simulink model "RobotRuka"  (R2020a)
settings: Solver=VariableStepAuto  StartTime=0.0  StopTime=10.0  RelTol=1e-3
values from neighbouring files (symbols this model uses):
  g = 9.81    [Podaci.m]
  Kd = 200    [Podaci.m]
  Kp = 900    [Podaci.m]
  lc1 = 0.8    [Podaci.m]
  m0 = m1*lc1*lc1+Il2    (= 6.5)    [Podaci.m]
  m1 = 10    [Podaci.m]
  m2 = 10    [Podaci.m]
libraries: fuzblock x2
settings Model: Creator=Aldin  LastModifiedBy=Aldin

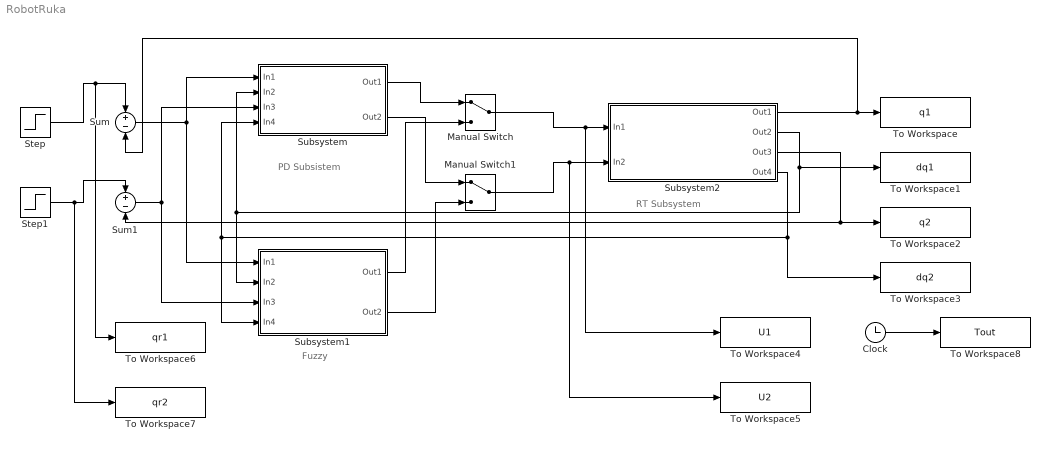
== system RobotRuka ==
  note: PD Subsistem
  note: Fuzzy
  note: RT Subsystem
  Clock : Clock
  Manual Switch : ManualSwitch
  Manual Switch1 : ManualSwitch
  Step : Step  Time=0  SampleTime=0
  Step1 : Step  Time=0  SampleTime=0
  Subsystem : Subsystem
  Subsystem1 : Subsystem
  Subsystem2 : Subsystem
  Sum : Sum  Inputs=+-
  Sum1 : Sum  Inputs=+-
  To Workspace : ToWorkspace  VariableName=q1  SampleTime=-1
  To Workspace1 : ToWorkspace  VariableName=dq1  SampleTime=-1
  To Workspace2 : ToWorkspace  VariableName=q2  SampleTime=-1
  To Workspace3 : ToWorkspace  VariableName=dq2  SampleTime=-1
  To Workspace4 : ToWorkspace  VariableName=U1  SampleTime=-1
  To Workspace5 : ToWorkspace  VariableName=U2  SampleTime=-1
  To Workspace6 : ToWorkspace  VariableName=qr1  SampleTime=-1
  To Workspace7 : ToWorkspace  VariableName=qr2  SampleTime=-1
  To Workspace8 : ToWorkspace  VariableName=Tout  SampleTime=-1
  wires:
  Subsystem2/4(Out4) -> Subsystem/4(In4), Subsystem1/4(In4), To Workspace3/1
  Subsystem1/2(Out2) -> Manual Switch1/2
  Clock/1 -> To Workspace8/1
  Manual Switch/1 -> To Workspace4/1, Subsystem2/1(In1)
  Subsystem2/1(Out1) -> To Workspace/1, Sum/2
  Subsystem1/1(Out1) -> Manual Switch/2
  Subsystem2/3(Out3) -> Sum1/2, To Workspace2/1
  Manual Switch1/1 -> To Workspace5/1, Subsystem2/2(In2)
  Sum1/1 -> Subsystem1/3(In3), Subsystem/3(In3)
  Subsystem2/2(Out2) -> To Workspace1/1, Subsystem1/2(In2), Subsystem/2(In2)
  Step1/1 -> To Workspace7/1, Sum1/1
  Sum/1 -> Subsystem/1(In1), Subsystem1/1(In1)
  Subsystem/1(Out1) -> Manual Switch/1
  Step/1 -> To Workspace6/1, Sum/1
  Subsystem/2(Out2) -> Manual Switch1/1

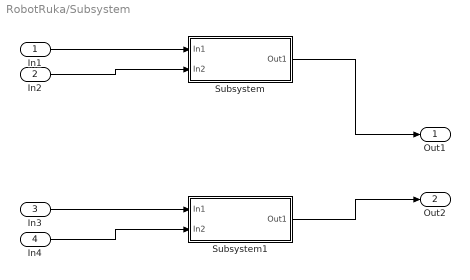
== system RobotRuka/Subsystem ==
  In1 : Inport
  In2 : Inport  Port=2
  In3 : Inport  Port=3
  In4 : Inport  Port=4
  Subsystem : Subsystem
  Subsystem1 : Subsystem
  Out1 : Outport
  Out2 : Outport  Port=2
  wires:
  Subsystem/1(Out1) -> Out1/1
  In1/1 -> Subsystem/1(In1)
  In2/1 -> Subsystem/2(In2)
  In3/1 -> Subsystem1/1(In1)
  In4/1 -> Subsystem1/2(In2)
  Subsystem1/1(Out1) -> Out2/1

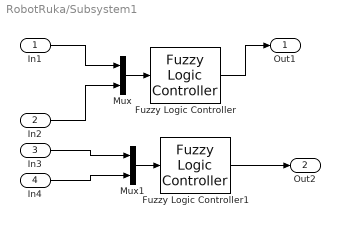
== system RobotRuka/Subsystem1 ==
  In1 : Inport
  In2 : Inport  Port=2
  In3 : Inport  Port=3
  In4 : Inport  Port=4
  Fuzzy Logic Controller : fuzblock/Fuzzy Logic  Controller  FIS=rtfuzzy  OutputSampleNumber=101  DataType=double  FuzzifiedInputs=off  RuleFiringStrengths=off  RuleOutputs=off  AggregatedOutputs=off  SimulateUsing=Interpreted execution  OutOfRangeInputValueMessage=warning  NoRuleFiredMessage=warning  EmptyOutputFuzzySetMessage=warning
  Fuzzy Logic Controller1 : fuzblock/Fuzzy Logic  Controller  FIS=rtfuzzy  OutputSampleNumber=101  DataType=double  FuzzifiedInputs=off  RuleFiringStrengths=off  RuleOutputs=off  AggregatedOutputs=off  SimulateUsing=Interpreted execution  OutOfRangeInputValueMessage=warning  NoRuleFiredMessage=warning  EmptyOutputFuzzySetMessage=warning
  Mux : Mux  Inputs=2
  Mux1 : Mux  Inputs=2
  Out1 : Outport
  Out2 : Outport  Port=2
  wires:
  Mux/1 -> Fuzzy Logic Controller/1
  In1/1 -> Mux/1
  In2/1 -> Mux/2
  Fuzzy Logic Controller/1 -> Out1/1
  Mux1/1 -> Fuzzy Logic Controller1/1
  In3/1 -> Mux1/1
  In4/1 -> Mux1/2
  Fuzzy Logic Controller1/1 -> Out2/1

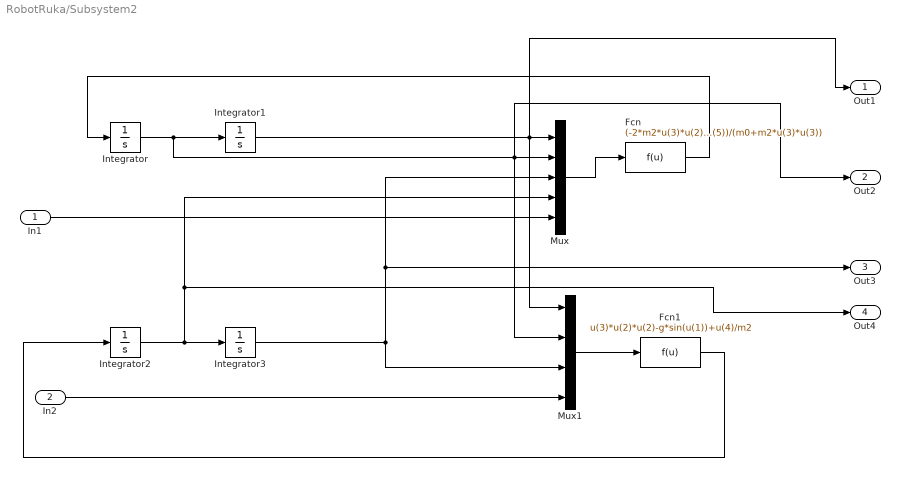
== system RobotRuka/Subsystem2 ==
  In1 : Inport
  In2 : Inport  Port=2
  Fcn : Fcn  Expr=(-2*m2*u(3)*u(2)*u(4)-m1*lc1*g*cos(u(1))-m2*g*u(3)*cos(u(1))+u(5))/(m0+m2*u(3)*u(3))
  Fcn1 : Fcn  Expr=u(3)*u(2)*u(2)-g*sin(u(1))+u(4)/m2
  Integrator{,1..3} (4 alike) : Integrator
  Mux : Mux  Inputs=5
  Mux1 : Mux
  Out1 : Outport
  Out2 : Outport  Port=2
  Out3 : Outport  Port=3
  Out4 : Outport  Port=4
  wires:
  In1/1 -> Mux/5
  Mux/1 -> Fcn/1
  Fcn/1 -> Integrator/1
  Integrator/1 -> Mux1/2, Out2/1, Mux/2, Integrator1/1
  Integrator1/1 -> Mux1/1, Out1/1, Mux/1
  Fcn1/1 -> Integrator2/1
  Integrator2/1 -> Out4/1, Mux/4, Integrator3/1
  Integrator3/1 -> Out3/1, Mux/3, Mux1/3
  In2/1 -> Mux1/4
  Mux1/1 -> Fcn1/1

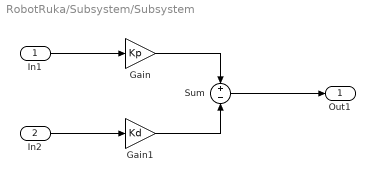
== system RobotRuka/Subsystem/Subsystem ==
  In1 : Inport
  In2 : Inport  Port=2
  Gain : Gain  Gain=Kp
  Gain1 : Gain  Gain=Kd
  Sum : Sum  Inputs=+-
  Out1 : Outport
  wires:
  Gain/1 -> Sum/1
  Gain1/1 -> Sum/2
  Sum/1 -> Out1/1
  In2/1 -> Gain1/1
  In1/1 -> Gain/1

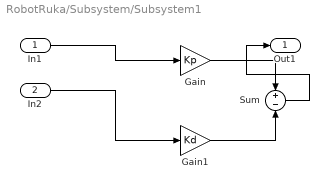
== system RobotRuka/Subsystem/Subsystem1 ==
  In1 : Inport
  In2 : Inport  Port=2
  Gain : Gain  Gain=Kp
  Gain1 : Gain  Gain=Kd
  Sum : Sum  Inputs=+-
  Out1 : Outport
  wires:
  Gain1/1 -> Sum/2
  Gain/1 -> Sum/1
  In1/1 -> Gain/1
  Sum/1 -> Out1/1
  In2/1 -> Gain1/1
